simulink model "C_rho"  (R2020a)
settings: Solver=VariableStepAuto  StartTime=0.0  StopTime=1  RelTol=1e-3
settings Model: Creator=Willie  LastModifiedBy=Willie

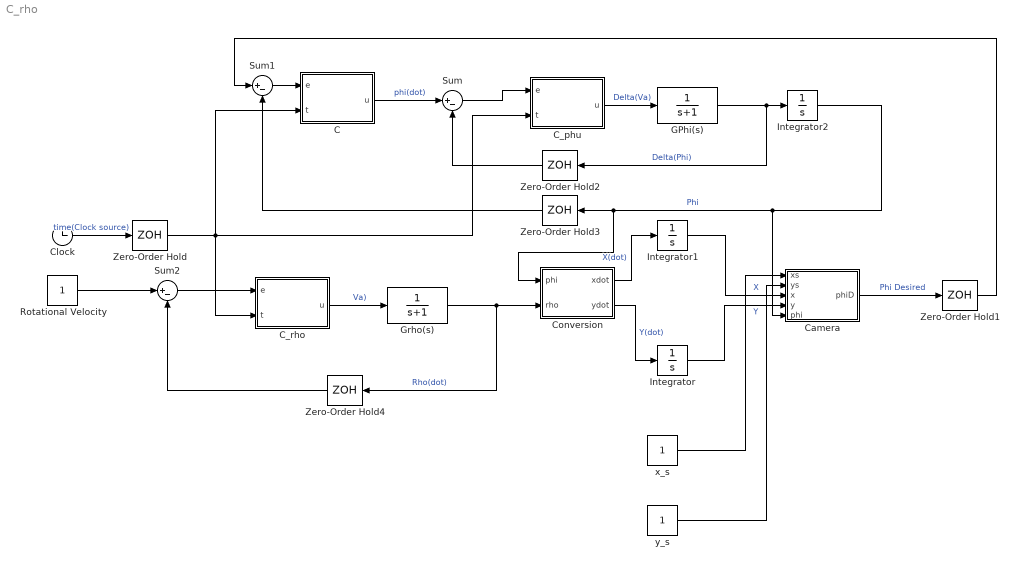
== system C_rho ==
  " GPhi(s)" : TransferFcn  Denominator=[1 1]
  C : MATLAB Function  TreatAsAtomicUnit=on
  C_phu : MATLAB Function  TreatAsAtomicUnit=on
  C_rho : MATLAB Function  TreatAsAtomicUnit=on
  Camera : MATLAB Function  TreatAsAtomicUnit=on
  Clock : Clock
  Conversion : MATLAB Function  TreatAsAtomicUnit=on
  Grho(s) : TransferFcn  Denominator=[1 1]
  Integrator : Integrator
  Integrator1 : Integrator
  Integrator2 : Integrator
  Rotational Velocity : Constant
  Sum : Sum  Inputs=|+-
  Sum1 : Sum  Inputs=|+-
  Sum2 : Sum  Inputs=|+-
  Zero-Order Hold{,1..4} (5 alike) : ZeroOrderHold  SampleTime=-1
  x_s : Constant
  y_s : Constant
  wires:
  Sum2/1 -> C_rho/1(e)
  Sum1/1 -> C/1(e)
  Clock/1 -> Zero-Order Hold/1  "time(Clock source)"
  Zero-Order Hold/1 -> C/2(t), C_phu/2(t), C_rho/2(t)
  C_rho/1(u) -> Grho(s)/1  "Va)"
  Grho(s)/1 -> Conversion/2(rho), Zero-Order Hold4/1  "Rho(dot)"
  Zero-Order Hold4/1 -> Sum2/2
  Rotational Velocity/1 -> Sum2/1
  C/1(u) -> Sum/1  "phi(dot)"
  Sum/1 -> C_phu/1(e)
  C_phu/1(u) -> " GPhi(s)"/1  "Delta(Va)"
  Zero-Order Hold2/1 -> Sum/2
  " GPhi(s)"/1 -> Integrator2/1, Zero-Order Hold2/1  "Delta(Phi)"
  Integrator2/1 -> Camera/5(phi), Zero-Order Hold3/1, Conversion/1(phi)  "Phi"
  Zero-Order Hold3/1 -> Sum1/2
  Conversion/1(xdot) -> Integrator1/1  "X(dot)"
  Conversion/2(ydot) -> Integrator/1  "Y(dot)"
  x_s/1 -> Camera/1(xs)
  y_s/1 -> Camera/2(ys)
  Integrator1/1 -> Camera/3(x)  "X"
  Integrator/1 -> Camera/4(y)  "Y"
  Camera/1(phiD) -> Zero-Order Hold1/1  "Phi Desired"
  Zero-Order Hold1/1 -> Sum1/1

== matlab function C_rho/C_phu ==
  data: e input; u output; t input
function u = fcn(e,t)
% Controller Gains
ki=1;
kp=1;
kd=1;
umax = 10;
%memory stuff
persistent I_past;
persistent t_past;
persistent e_past;
if isempty(I_past), I_past=0; end;
if isempty(t_past), t_past=0; end;
if isempty(e_past), e_past=0; end;
%controller calculations
Ts=t-t_past; %sample time
I=I_past+e*Ts; %integrator
D=(e-e_past)/Ts; % Derivative
u=kp*e+ki*I+kd*D; % PID controller Equation

if(abs(u)>umax)
u=sign(u)*umax;
e=sign(e)*min(umax/kp,abs(e));
I=(u-kp*e-kd*D)/ki;
end;
I_past=I;
t_past=t;
e_past=e;

== matlab function C_rho/Conversion ==
  data: xdot output; ydot output; phi input; rho input
function [xdot,ydot]= fcn(phi, rho)

xdot=phi*cos(rho);
ydot=phi*sin(rho);

== matlab function C_rho/C ==
  data: e input; u output; t input
function u = fcn(e,t)
% Controller Gains
ki=1;
kp=1;
kd=1;
umax = 10;
%memory stuff
persistent I_past;
persistent t_past;
persistent e_past;
if isempty(I_past), I_past=0; end;
if isempty(t_past), t_past=0; end;
if isempty(e_past), e_past=0; end;
%controller calculations
Ts=t-t_past; %sample time
I=I_past+e*Ts; %integrator
D=(e-e_past)/Ts; % Derivative
u=kp*e+ki*I+kd*D; % PID controller Equation

if(abs(u)>umax)
u=sign(u)*umax;
e=sign(e)*min(umax/kp,abs(e));
I=(u-kp*e-kd*D)/ki;
end;
I_past=I;
t_past=t;
e_past=e;

== matlab function C_rho/C_rho ==
  data: e input; u output; t input
function u = fcn(e,t)
% Controller Gains
ki=1;
kp=1;
kd=1;
umax = 10;
%memory stuff
persistent I_past;
persistent t_past;
persistent e_past;
if isempty(I_past), I_past=0; end;
if isempty(t_past), t_past=0; end;
if isempty(e_past), e_past=0; end;
%controller calculations
Ts=t-t_past; %sample time
I=I_past+e*Ts; %integrator
D=(e-e_past)/Ts; % Derivative
u=kp*e+ki*I+kd*D; % PID controller Equation

if(abs(u)>umax)
u=sign(u)*umax;
e=sign(e)*min(umax/kp,abs(e));
I=(u-kp*e-kd*D)/ki;
end;
I_past=I;
t_past=t;
e_past=e;

== matlab function C_rho/Camera ==
  data: xs input; phiD output; ys input; x input; y input; phi input
function phiD = fcn(xs,ys,x,y,phi)

phiD=phi+atan2(ys-y,xs-x)-phi; % not 100% on the - phi at the end becuase it counters our actual phi, they maybe differing Phi values
